simulink model "hw5"  (R2018b)
settings: Solver=FixedStepAuto  StartTime=0.0  StopTime=10.0  FixedStep=1e-3  RelTol=1e-3
values from neighbouring files (symbols this model uses):
  yo = 1    [MAIN_hw5.m]
settings Model: Creator=Erivelton  LastModifiedBy=Erivelton

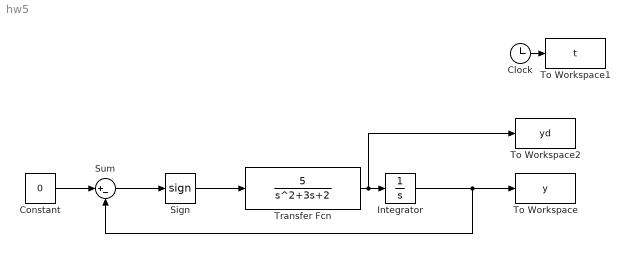
== system hw5 ==
  Clock : Clock
  Constant : Constant  Value=0
  Integrator : Integrator  InitialCondition=yo
  Sign : Signum
  Sum : Sum  Inputs=|+-
  To Workspace : ToWorkspace  VariableName=y  SampleTime=-1
  To Workspace1 : ToWorkspace  VariableName=t  SampleTime=-1
  To Workspace2 : ToWorkspace  VariableName=yd  SampleTime=-1
  Transfer Fcn : TransferFcn  Numerator=[5]  Denominator=[1 3 2]
  wires:
  Sum/1 -> Sign/1
  Sign/1 -> Transfer Fcn/1
  Transfer Fcn/1 -> To Workspace2/1, Integrator/1
  Constant/1 -> Sum/1
  Clock/1 -> To Workspace1/1
  Integrator/1 -> Sum/2, To Workspace/1
